simulink model "motorcc_fuzzy"  (R2021b)
settings: Solver=VariableStepAuto  StartTime=0.0  StopTime=4  RelTol=1e-3
libraries: fuzblock x1, simulink_extras x1
settings Model: Creator=Usuario_UMA  LastModifiedBy=Daniel
settings SolverCC: AlgebraicLoopSolver=TrustRegion
settings DebuggingCC: SFMachineParentedDataDiag=warning

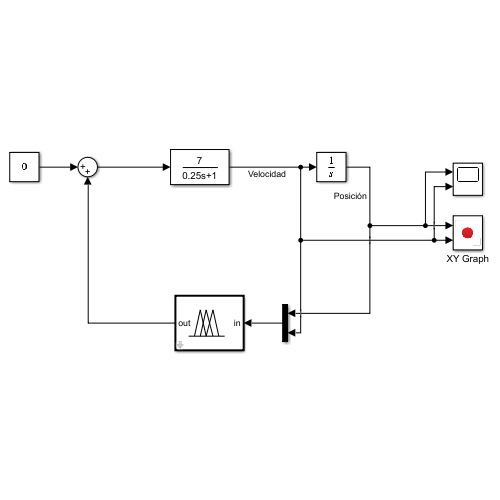
[thumbnail: Simulink's stored preview of the top-level diagram]
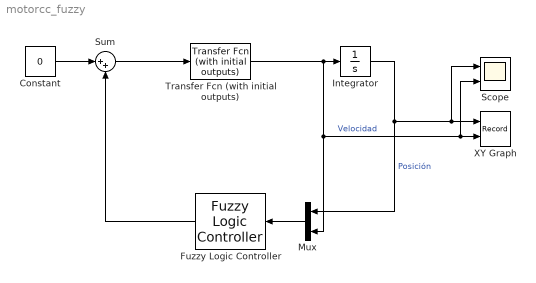
== system motorcc_fuzzy ==
  Constant : Constant  Value=0
  Fuzzy Logic Controller : fuzblock/Fuzzy Logic  Controller  FIS=FIS3  OutputSampleNumber=101  DataType=double  FuzzifiedInputs=off  RuleFiringStrengths=off  RuleOutputs=off  AggregatedOutputs=off  SimulateUsing=Interpreted execution  OutOfRangeInputValueMessage=warning  NoRuleFiredMessage=warning  EmptyOutputFuzzySetMessage=warning
  Integrator : Integrator  InitialCondition=3
  Mux : Mux  Inputs=2
  Scope : Scope  NumInputPorts=2
  Sum : Sum  Inputs=|++
  Transfer Fcn (with initial outputs) : simulink_extras/Additional Linear/Transfer Fcn (with initial outputs)  N=[7]  D="[0.25  1]"  Y0=0.5  U0=0
  XY Graph : Record  FileSettingsInternal="{\"entries\":[{\"content\":{\"excelSettings\":{\"content\":{},\"type\":\"Streamout.ExcelSettings\"}},\"type\":\"Streamout.FileSettingStorage\",\"uuid\":\"db02bd41-e65a-46fd-bbd6-a3364cef3c3f\"}],\"packageUris\":[\"http://schema.mathworks.com/mf0/streamout_blocks/R2020a\"],\"version\":\"1.0\"}"  Layout=[1 1]  SignalsInternal="{\"entries\":[{\"content\":{\"signals\":[{\"content\":{\"blockPath\":[\"motorcc_fuzzy/XY Graph\"],\"channel\":[],\"dimensions\":[1],\"domain\":\"motorcc_fuzzy/XY Graph\",\"lineColor\":\"#a2142f\",\"plots\":[1],\"port\":1,\"sid\":[\"\"],\"signalID\":8720,\"signalName\":\"Posición\"},\"type\":\"RecordBlkView.Signal\",\"uuid\":\"5fea4636-605e-450f-8da4-770a367e6e2f\"},{\"content\":{\"blockPath\":[\"motorcc_fuzzy/XY Graph\"],\"channel\":[],\"dimensions\":[1],\"domain\":\"motorcc_fuzzy/XY Graph\",\"lineColor\":\"#139fff\",\"plots\":[1],\"port\":2,\"sid\":[\"\"],\"signalID\":8724,\"signalName\":\"Velocidad\"},\"type\":\"RecordBlkView.Signal\",\"uuid\":\"478a0676-9306-43ce-b7e6-4e0b12ecf515\"}]},\"type\":\"RecordBlkView.InputSignals\",\"uuid\":\"935c0e1a-8eec-4e26-b260-239be53949f8\"}],\"packageUris\":[\"http://schema.mathworks.com/mf0/streamout_blocks/R2020a\"],\"version\":\"1.0\"}"  VisualizationBindings="{\"xyplotplugin\":{\"info\":[{\"series\":[{\"bindingParametersList\":[{\"parameter\":\"X-Axis\",\"signalID\":8720,\"signalName\":\"PosiciÃ³n\"},{\"parameter\":\"Y-Axis\",\"signalID\":8724,\"signalName\":\"Velocidad\"}],\"seriesID\":42952}],\"subplotID\":1}]}}"  CompatibilityTag=XY  st=-1
  wires:
  Transfer Fcn (with initial outputs)/1 -> Scope/2, XY Graph/2, Mux/2, Integrator/1  "Velocidad"
  Mux/1 -> Fuzzy Logic Controller/1
  Integrator/1 -> XY Graph/1, Scope/1, Mux/1  "Posición"
  Sum/1 -> Transfer Fcn (with initial outputs)/1
  Fuzzy Logic Controller/1 -> Sum/2
  Constant/1 -> Sum/1
